simulink model "P3_Ex12aNOISE"  (R2018a)
settings: Solver=FixedStepAuto  StartTime=0.0  StopTime=10  RelTol=1e-3  EnableMultiTasking=on
PreLoadFcn:
  | % Plant
  | K0=0.82/0.017;
  | tau0=0.26;
  | N=9;
  | Kpot=1.62;
  | % Sampling period
  | Ts=0.01;
  | 
  | % Desired control specifications
  | Sp=80; % overshoot
  | Fd=0.5; % frequency
  | 
  | % Poles of the second order continuous system that will fulfill the specifications
  | wd=2*pi*Fd ;
  | xi=sqrt((log(Sp/100))^2/(pi^2+log(Sp/100)^2))
  | wn=wd/ sqrt(1-xi^2)
  | s1=-xi*wn+j*wd
  | s2=-xi*wn-j*wd
  | 
  | % Poles of the second order discrete system that will fulfill the specifications
  | p1=exp(Ts* s1 )
  | p2=exp(Ts* s2 )
  | % Fix third pole
  | p3=0.01
  | 
  | % Plant's Z transfere function
  | Ptas=tf([K0*(1/N)*Kpot],[tau0,1,0]);
  | Ptaz=c2d(Ptas,Ts,'zoh');
  | 
  | % Denominator and numerator coefficients
  | [Nz ,Dz]= tfdata(Ptaz,'v')
  | a1=Nz(2);
  | a0=Nz(3);
  | b1=Dz(2);
  | b0=Dz(3);
  | 
  | % A and B matrix definitions
  | A=[-1 -a1 -a1 -a1 ; p2+p3+p1 a1-a0 -a1-a0 -a0+2*a1 ; ...
  |    -p1*p2-p3*p1-p2*p3 a0 -a0 2*a0-a1 ; p1*p2*p3 0 0 -a0 ] ;
  | b=[p1+p2+p3-1+b1 ; -p1*p2-p3*p1-p3*p2+b0-b1 ; p1*p2*p3-b0 ; 0 ] ;
  | 
  | % x vector's determination of the controller
  | x=inv(A)*b ;
  | 
  | p4=x(1)
  | Kp=x(2)
  | Ki=(2/Ts)*x(3)
  | Kd=Ts*x(4)
  | pawd=0.2;
  | Kaw=1/Ki;
  | 
  | % Poles dominance calculation
  | dominancia=log(abs(p4))/log(abs(p1))
undefined symbols (not defined in the file or in its folder): DiscIntNeverNeededParam
libraries: simulink x2
settings Model: ExtModeTrigDuration=2  Creator=Eneko Lerma  LastModifiedBy=Eneko Lerma
settings OptimizationCC: EnhancedBackFolding=on  PassReuseOutputArgsAs=Individual arguments  MaxStackSize=64  OptimizeBlockOrder=speed  DifferentSizesBufferReuse=on  OptimizationCustomize=off
settings DebuggingCC: ParameterPrecisionLossMsg=none  ParameterTunabilityLossMsg=error
settings HardwareCC: ProdBitPerPointer=32  ProdBitPerSizeT=32  ProdBitPerPtrDiffT=32  ProdLargestAtomicInteger=Long  ProdLargestAtomicFloat=Double  ProdWordSize=32  ProdHWDeviceType=ARM Compatible->ARM Cortex
settings SFSimCC: MATLABDynamicMemAlloc=off
settings RTWCC: SystemTargetFile=ert.tlc  HardwareBoard=Arduino Due  TLCOptions=-aInlineSetEventsForThisBaseRateFcn=TLC_FALSE -aSuppressMultiTaskScheduler=TLC_FALSE -aRateBasedStepFcn=1  TemplateMakefile=ert_default_tmf  GenerateReport=on  Toolchain=Arduino ARM  BuildConfiguration=Faster Runs  IncludeHyperlinkInReport=on  LaunchReport=on  GenerateTraceInfo=on  GenerateTraceReport=on  GenerateTraceReportSl=on  GenerateTraceReportSf=on  GenerateTraceReportEml=on
settings CodeAppCC: ForceParamTrailComments=on  IgnoreCustomStorageClasses=off  OperatorAnnotations=on  SimulinkDataObjDesc=on  SFDataObjDesc=on  InsertBlockDesc=on
settings ERTTargetCC: SupportContinuousTime=on  SupportVariableSizeSignals=on

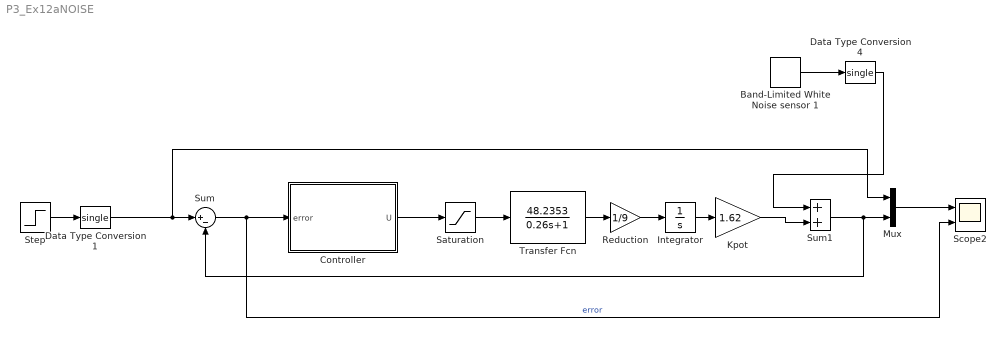
== system P3_Ex12aNOISE ==
  Band-Limited White Noise sensor 1 : simulink/Sources/Band-Limited White Noise  Cov=[0.00002]  Ts=0.01  seed=[23341]
  Controller : Subsystem
  Data Type Conversion1 : DataTypeConversion  OutDataTypeStr=single
  Data Type Conversion4 : DataTypeConversion  OutDataTypeStr=single
  Integrator : Integrator
  Kpot : Gain  Gain=1.62  OutDataTypeStr=single
  Mux : Mux  Inputs=2
  Reduction : Gain  Gain=1/9  OutDataTypeStr=double
  Saturation : Saturate  UpperLimit=5  LowerLimit=-5  OutDataTypeStr=double
  Scope2 : Scope  NumInputPorts=2
  Step : Step  Time=0  SampleTime=0
  Sum : Sum  Inputs=|+-  AccumDataTypeStr=single
  Sum1 : Sum
  Transfer Fcn : TransferFcn  Numerator=[48.2353]  Denominator=[0.26 1]
  wires:
  Mux/1 -> Scope2/1
  Step/1 -> Data Type Conversion1/1
  Kpot/1 -> Sum1/2
  Data Type Conversion1/1 -> Sum/1, Mux/1
  Sum/1 -> Scope2/2, Controller/1(error)  "error"
  Saturation/1 -> Transfer Fcn/1
  Transfer Fcn/1 -> Reduction/1
  Reduction/1 -> Integrator/1
  Integrator/1 -> Kpot/1
  Controller/1(U) -> Saturation/1
  Band-Limited White Noise sensor 1/1 -> Data Type Conversion4/1
  Data Type Conversion4/1 -> Sum1/1
  Sum1/1 -> Sum/2, Mux/2

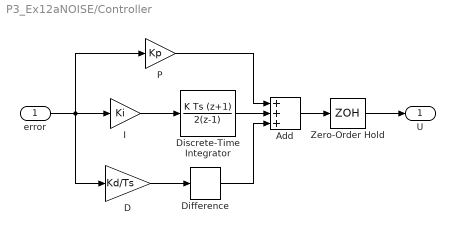
== system P3_Ex12aNOISE/Controller ==
  error : Inport
  Add : Sum  Inputs=+++  AccumDataTypeStr=single
  D : Gain  Gain=Kd/Ts
  Difference : simulink/Discrete/Difference  ICPrevInput=0.0  OutMin=[]  OutMax=[]  OutDataType=fixdt(1, 16)  OutScaling=2^-10  DoSatur=off
  Discrete-Time Integrator : DiscreteIntegrator  IntegratorMethod=Integration: Trapezoidal  SampleTime=Ts  ICPrevOutput=DiscIntNeverNeededParam  ICPrevScaledInput=DiscIntNeverNeededParam
  I : Gain  Gain=Ki
  P : Gain  Gain=Kp
  Zero-Order Hold : ZeroOrderHold  SampleTime=Ts
  U : Outport
  wires:
  Difference/1 -> Add/3
  Discrete-Time Integrator/1 -> Add/2
  Add/1 -> Zero-Order Hold/1
  error/1 -> P/1, I/1, D/1
  I/1 -> Discrete-Time Integrator/1
  P/1 -> Add/1
  D/1 -> Difference/1
  Zero-Order Hold/1 -> U/1
